simulink model "CSEI_HIL"  (R2020b)
settings: Solver=FixedStepAuto  StartTime=0.0  StopTime=Inf  FixedStep=0.01  RelTol=1e-3  EnableMultiTasking=on
undefined symbols (not defined in the file): X, Y, Z
libraries: robotlib x6, simulink x3
settings Model: Creator=erlendbasso  LastModifiedBy=erlendbasso
settings SolverCC: PositivePriorityOrder=on
settings OptimizationCC: EnhancedBackFolding=on  PassReuseOutputArgsAs=Individual arguments  ZeroExternalMemoryAtStartup=off  ZeroInternalMemoryAtStartup=off  MaxStackSize=64  OptimizeBlockOrder=speed  DifferentSizesBufferReuse=on  OptimizationCustomize=off  EfficientTunableParamExpr=on
settings DebuggingCC: ParameterTunabilityLossMsg=error
settings HardwareCC: ProdBitPerPointer=32  ProdBitPerSizeT=32  ProdBitPerPtrDiffT=32  ProdLargestAtomicInteger=Long  ProdLargestAtomicFloat=Double  ProdWordSize=32  ProdHWDeviceType=ARM Compatible->ARM Cortex
settings RTWCC: Description=Embedded Coder  SystemTargetFile=ert.tlc  HardwareBoard=Raspberry Pi - Robot Operating System (ROS)  TLCOptions="-aInlineSetEventsForThisBaseRateFcn=TLC_FALSE -aSuppressMultiTaskScheduler=TLC_FALSE  -aRateBasedStepFcn=0"  TemplateMakefile=ert_default_tmf  Toolchain=Catkin  TargetLang=C++
settings CodeAppCC: ForceParamTrailComments=on  IgnoreCustomStorageClasses=off  OperatorAnnotations=on  SimulinkDataObjDesc=on  SFDataObjDesc=on  InsertBlockDesc=on
settings ERTTargetCC: SupportContinuousTime=on

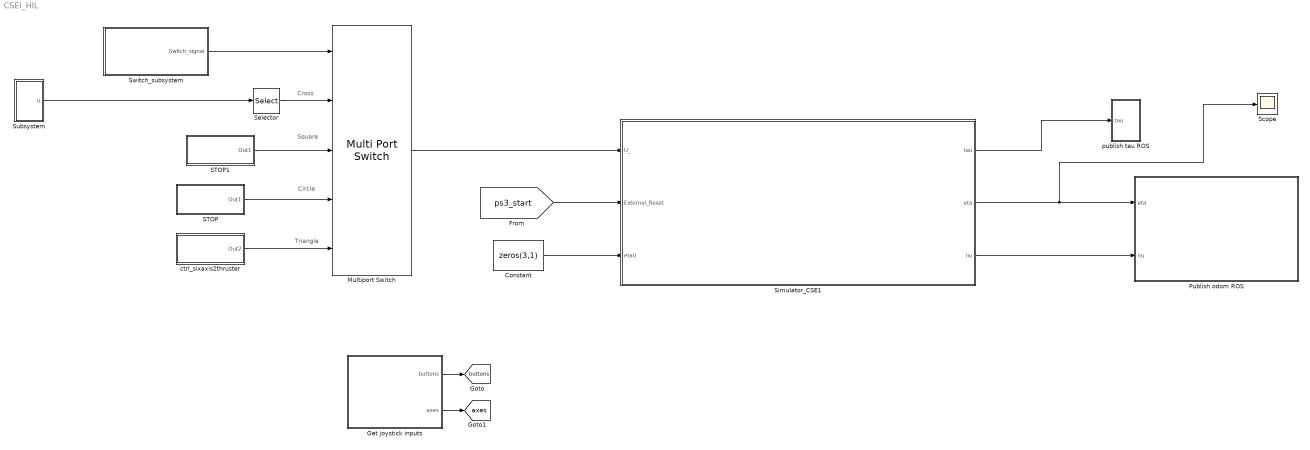
== system CSEI_HIL ==
  note: Square
  note: Triangle
  note: Circle
  note: Cross
  Constant : Constant  Value=zeros(3,1)
  Get joystick inputs : Subsystem
  Multiport Switch : MultiPortSwitch  Inputs=4
  Publish odom ROS : Subsystem
  STOP : Subsystem
  STOP1 : Subsystem
  Scope : Scope
  Selector : Selector  InputPortWidth=128  IndexOptions=Index vector (dialog)  Indices=[1:5]  OutputSizes=1
  Simulator_CSE1 : Subsystem
  Subsystem : Subsystem
  Switch_subsystem : Subsystem
  ctrl_sixaxis2thruster : Subsystem
  publish tau ROS : Subsystem
  tag scope: axes=global, buttons=global
  wires:
  Subsystem/1(u) -> Selector/1
  Switch_subsystem/1(Switch_signal) -> Multiport Switch/1
  ctrl_sixaxis2thruster/1(Out2) -> Multiport Switch/5
  STOP1/1(Out1) -> Multiport Switch/3
  STOP/1(Out1) -> Multiport Switch/4
  Get joystick inputs/1(buttons) -> [buttons]
  Get joystick inputs/2(axes) -> [axes]
  Constant/1 -> Simulator_CSE1/3(eta0)
  Simulator_CSE1/1(tau) -> publish tau ROS/1(tau)
  Simulator_CSE1/2(eta) -> Scope/1, Publish odom ROS/1(eta)
  Simulator_CSE1/3(nu) -> Publish odom ROS/2(nu)
  [ps3_start] -> Simulator_CSE1/2(External_Reset)
  Multiport Switch/1 -> Simulator_CSE1/1(U_)
  Selector/1 -> Multiport Switch/2

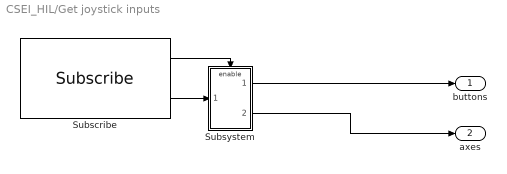
== system CSEI_HIL/Get joystick inputs ==
  Subscribe : robotlib/Subscribe  topicSource=Specify your own  topic=/joy  messageType=sensor_msgs/Joy  SampleTime=0.01  legacyBusStruct=off  messageQueueLength=1
  Subsystem : Subsystem
  buttons : Outport
  axes : Outport  Port=2
  wires:
  Subscribe/1 -> Subsystem/Enable
  Subscribe/2 -> Subsystem/1(In1)
  Subsystem/1(<Buttons>) -> buttons/1
  Subsystem/2(<Axes>) -> axes/1

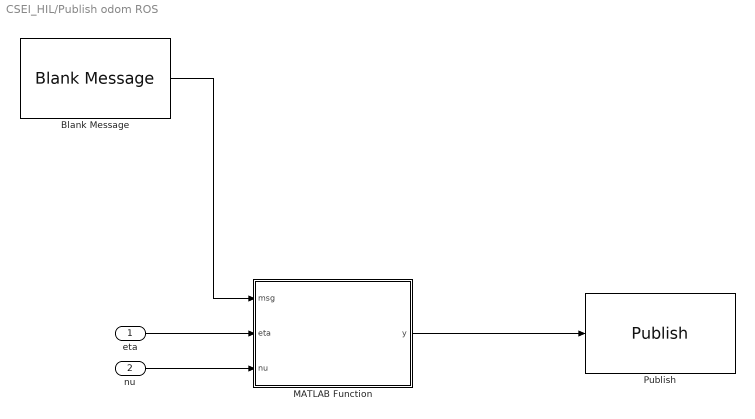
== system CSEI_HIL/Publish odom ROS ==
  eta : Inport
  nu : Inport  Port=2
  Blank Message : robotlib/Blank Message  messageClass=Message  entityType=nav_msgs/Odometry  messageType=nav_msgs/Odometry  SampleTime=0.01  legacyBusStruct=off
  MATLAB Function : MATLAB Function  TreatAsAtomicUnit=on
  Publish : robotlib/Publish  topicSource=Specify your own  topic=/qualisys/CSEI/odom  messageType=nav_msgs/Odometry  legacyBusStruct=off  messageQueueLength=1
  wires:
  MATLAB Function/1(y) -> Publish/1
  Blank Message/1 -> MATLAB Function/1(msg)
  eta/1 -> MATLAB Function/2(eta)
  nu/1 -> MATLAB Function/3(nu)

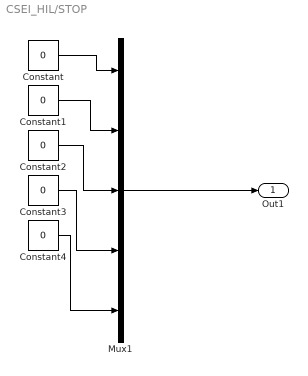
== system CSEI_HIL/STOP ==
  Constant{,1..4} (5 alike) : Constant  Value=0
  Mux1 : Mux  Inputs=5
  Out1 : Outport
  wires:
  Mux1/1 -> Out1/1
  Constant/1 -> Mux1/1
  Constant1/1 -> Mux1/2
  Constant2/1 -> Mux1/3
  Constant3/1 -> Mux1/4
  Constant4/1 -> Mux1/5

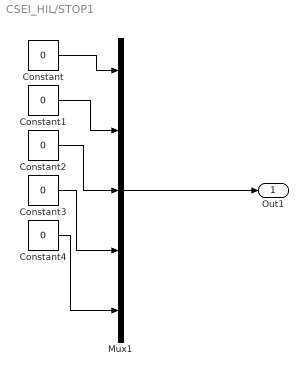
== system CSEI_HIL/STOP1 ==
  Constant{,1..4} (5 alike) : Constant  Value=0
  Mux1 : Mux  Inputs=5
  Out1 : Outport
  wires:
  Mux1/1 -> Out1/1
  Constant/1 -> Mux1/1
  Constant1/1 -> Mux1/2
  Constant2/1 -> Mux1/3
  Constant3/1 -> Mux1/4
  Constant4/1 -> Mux1/5

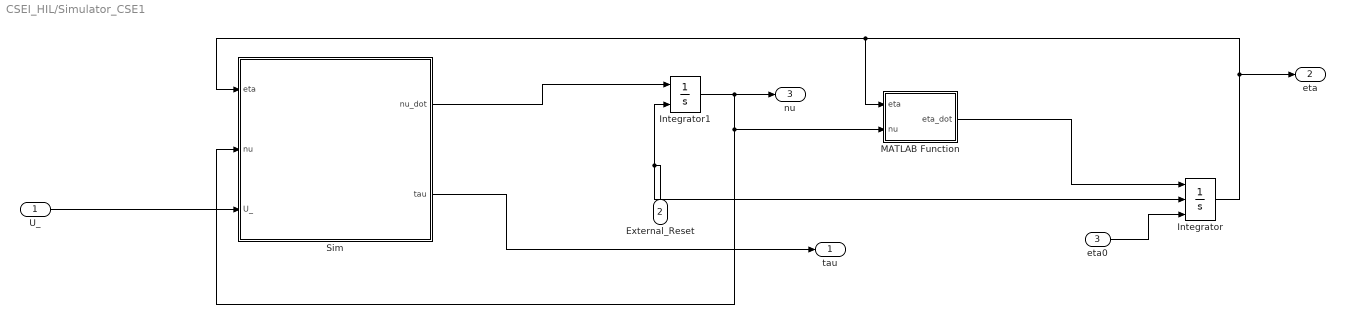
== system CSEI_HIL/Simulator_CSE1 ==
  U_ : Inport
  External_Reset : Inport  Port=2
  eta0 : Inport  Port=3
  Integrator : Integrator  ExternalReset=rising  InitialConditionSource=external  WrapState=on  WrappedStateUpperValue=[Inf;inf;pi]  WrappedStateLowerValue=[-Inf;-Inf;-pi]
  Integrator1 : Integrator  ExternalReset=rising  InitialCondition=zeros(3,1)
  MATLAB Function : MATLAB Function  TreatAsAtomicUnit=on
  Sim : MATLAB Function  TreatAsAtomicUnit=on
  tau : Outport
  eta : Outport  Port=2
  nu : Outport  Port=3
  wires:
  U_/1 -> Sim/3(U_)
  eta0/1 -> Integrator/3
  Sim/1(nu_dot) -> Integrator1/1
  External_Reset/1 -> Integrator/2, Integrator1/2
  Integrator1/1 -> MATLAB Function/2(nu), Sim/2(nu), nu/1
  Integrator/1 -> Sim/1(eta), MATLAB Function/1(eta), eta/1
  Sim/2(tau) -> tau/1
  MATLAB Function/1(eta_dot) -> Integrator/1

== system CSEI_HIL/Subsystem ==
  Bus Selector1 : BusSelector  OutputSignals=Data
  Subscribe : robotlib/Subscribe  topicSource=Specify your own  topic=/CSEI/u  messageType=std_msgs/Float64MultiArray  SampleTime=0.01  legacyBusStruct=off  messageQueueLength=1
  Subsystem1 : Subsystem
  u : Outport
  wires:
  Subscribe/1 -> Subsystem1/Enable
  Subscribe/2 -> Bus Selector1/1
  Subsystem1/1(Out1) -> u/1
  Bus Selector1/1 -> Subsystem1/1(<data>)  "<Data>"

== system CSEI_HIL/Switch_subsystem ==
  Memory : Memory  InitialCondition=4
  Switch_function : MATLAB Function  TreatAsAtomicUnit=on
  Switch_signal : Outport
  wires:
  Memory/1 -> Switch_function/2(temp)
  Switch_function/1(switch_signal) -> Switch_signal/1, Memory/1
  [buttons] -> Switch_function/1(buttons)

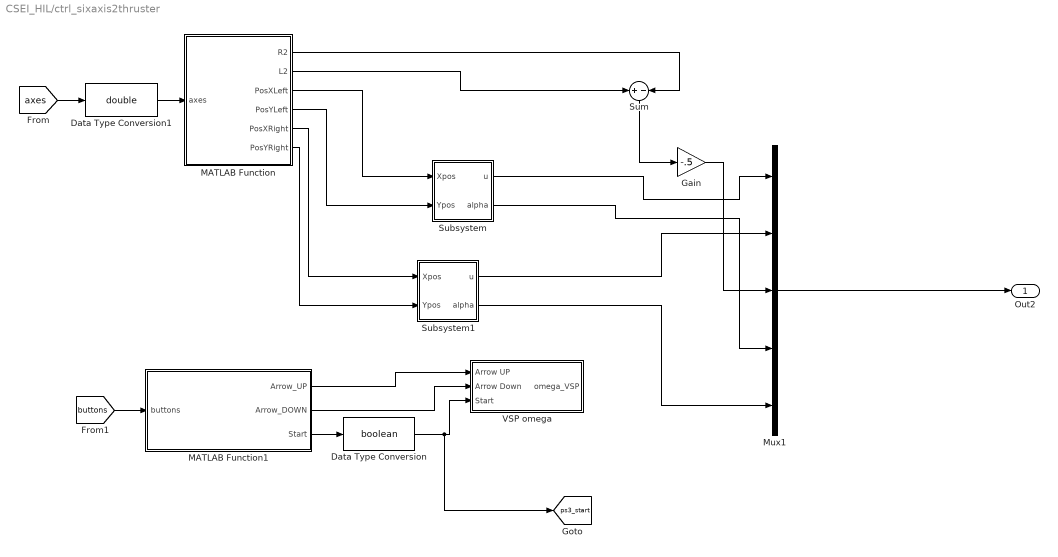
== system CSEI_HIL/ctrl_sixaxis2thruster ==
  Data Type Conversion : DataTypeConversion  OutDataTypeStr=boolean
  Data Type Conversion1 : DataTypeConversion  OutDataTypeStr=double
  Gain : Gain  Gain=-.5
  MATLAB Function : MATLAB Function  TreatAsAtomicUnit=on
  MATLAB Function1 : MATLAB Function  TreatAsAtomicUnit=on
  Mux1 : Mux  Inputs=5
  Subsystem : Subsystem
  Subsystem1 : Subsystem
  Sum : Sum  Inputs=+|-
  VSP omega : Subsystem
  Out2 : Outport
  tag scope: ps3_start=global
  wires:
  Mux1/1 -> Out2/1
  Subsystem/2(alpha) -> Mux1/4
  Subsystem1/2(alpha) -> Mux1/5
  MATLAB Function/1(R2) -> Sum/2
  Sum/1 -> Gain/1
  MATLAB Function/2(L2) -> Sum/1
  [axes] -> Data Type Conversion1/1
  MATLAB Function/3(PosXLeft) -> Subsystem/1(Xpos)
  MATLAB Function/4(PosYLeft) -> Subsystem/2(Ypos)
  MATLAB Function/5(PosXRight) -> Subsystem1/1(Xpos)
  MATLAB Function/6(PosYRight) -> Subsystem1/2(Ypos)
  [buttons] -> MATLAB Function1/1(buttons)
  MATLAB Function1/1(Arrow_UP) -> VSP omega/1(Arrow UP)
  MATLAB Function1/2(Arrow_DOWN) -> VSP omega/2(Arrow Down)
  MATLAB Function1/3(Start) -> Data Type Conversion/1
  Data Type Conversion/1 -> [ps3_start], VSP omega/3(Start)
  Data Type Conversion1/1 -> MATLAB Function/1(axes)
  Subsystem/1(u) -> Mux1/1
  Subsystem1/1(u) -> Mux1/2
  Gain/1 -> Mux1/3

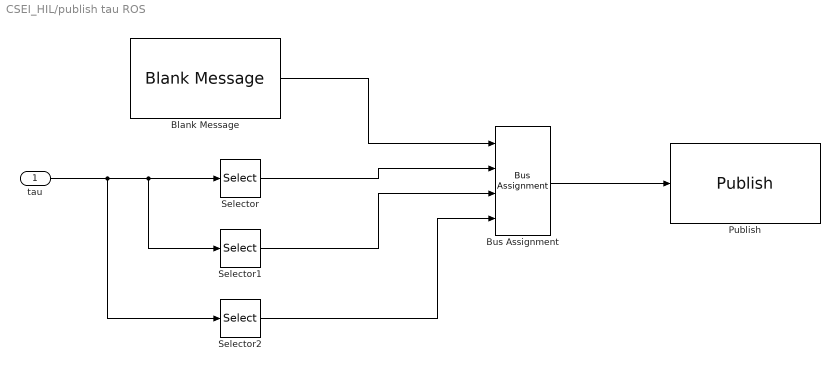
== system CSEI_HIL/publish tau ROS ==
  tau : Inport
  Blank Message : robotlib/Blank Message  messageClass=Message  entityType=geometry_msgs/Vector3  messageType=geometry_msgs/Vector3  SampleTime=0.01  legacyBusStruct=off
  Bus Assignment : BusAssignment  AssignedSignals=X,Y,Z
  Publish : robotlib/Publish  topicSource=Specify your own  topic=/CSEI/tau  messageType=geometry_msgs/Vector3  legacyBusStruct=off  messageQueueLength=1
  Selector : Selector  InputPortWidth=3  IndexOptions=Index vector (dialog)  Indices=[1]  OutputSizes=1
  Selector1 : Selector  InputPortWidth=3  IndexOptions=Index vector (dialog)  Indices=[2]  OutputSizes=1
  Selector2 : Selector  InputPortWidth=3  IndexOptions=Index vector (dialog)  Indices=[3]  OutputSizes=1
  wires:
  Bus Assignment/1 -> Publish/1
  Blank Message/1 -> Bus Assignment/1
  tau/1 -> Selector2/1, Selector1/1, Selector/1
  Selector/1 -> Bus Assignment/2
  Selector1/1 -> Bus Assignment/3
  Selector2/1 -> Bus Assignment/4

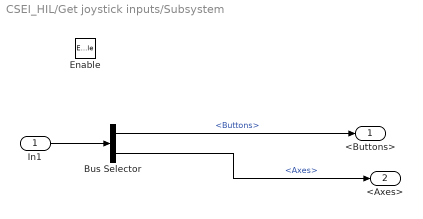
== system CSEI_HIL/Get joystick inputs/Subsystem ==
  In1 : Inport
  Enable : EnablePort
  Bus Selector : BusSelector  OutputSignals=Buttons,Axes
  <Buttons> : Outport
  <Axes> : Outport  Port=2
  wires:
  In1/1 -> Bus Selector/1
  Bus Selector/1 -> <Buttons>/1  "<Buttons>"
  Bus Selector/2 -> <Axes>/1  "<Axes>"

== system CSEI_HIL/Subsystem/Subsystem1 ==
  <data> : Inport
  Enable : EnablePort
  Bus to Vector : BusToVector
  Out1 : Outport
  wires:
  Bus to Vector/1 -> Out1/1
  <data>/1 -> Bus to Vector/1

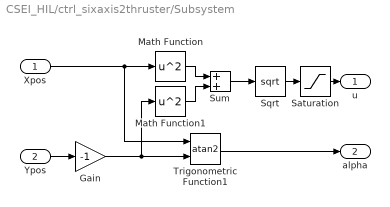
== system CSEI_HIL/ctrl_sixaxis2thruster/Subsystem ==
  Xpos : Inport
  Ypos : Inport  Port=2
  Gain : Gain  Gain=-1
  Math Function : Math  Operator=square  SignedPower=on  SaturateOnIntegerOverflow=on
  Math Function1 : Math  Operator=square  SignedPower=on  SaturateOnIntegerOverflow=on
  Saturation : Saturate  UpperLimit=1  LowerLimit=-1
  Sqrt : Sqrt  SaturateOnIntegerOverflow=on
  Sum : Sum
  Trigonometric Function1 : Trigonometry  Operator=atan2
  u : Outport
  alpha : Outport  Port=2
  wires:
  Xpos/1 -> Math Function/1, Trigonometric Function1/1
  Gain/1 -> Math Function1/1, Trigonometric Function1/2
  Trigonometric Function1/1 -> alpha/1
  Ypos/1 -> Gain/1
  Sum/1 -> Sqrt/1
  Math Function/1 -> Sum/1
  Math Function1/1 -> Sum/2
  Sqrt/1 -> Saturation/1
  Saturation/1 -> u/1

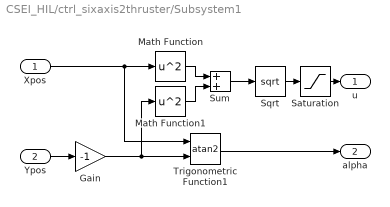
== system CSEI_HIL/ctrl_sixaxis2thruster/Subsystem1 ==
  Xpos : Inport
  Ypos : Inport  Port=2
  Gain : Gain  Gain=-1
  Math Function : Math  Operator=square  SignedPower=on  SaturateOnIntegerOverflow=on
  Math Function1 : Math  Operator=square  SignedPower=on  SaturateOnIntegerOverflow=on
  Saturation : Saturate  UpperLimit=1  LowerLimit=-1
  Sqrt : Sqrt  SaturateOnIntegerOverflow=on
  Sum : Sum
  Trigonometric Function1 : Trigonometry  Operator=atan2
  u : Outport
  alpha : Outport  Port=2
  wires:
  Xpos/1 -> Math Function/1, Trigonometric Function1/1
  Gain/1 -> Math Function1/1, Trigonometric Function1/2
  Trigonometric Function1/1 -> alpha/1
  Ypos/1 -> Gain/1
  Sum/1 -> Sqrt/1
  Math Function/1 -> Sum/1
  Math Function1/1 -> Sum/2
  Sqrt/1 -> Saturation/1
  Saturation/1 -> u/1

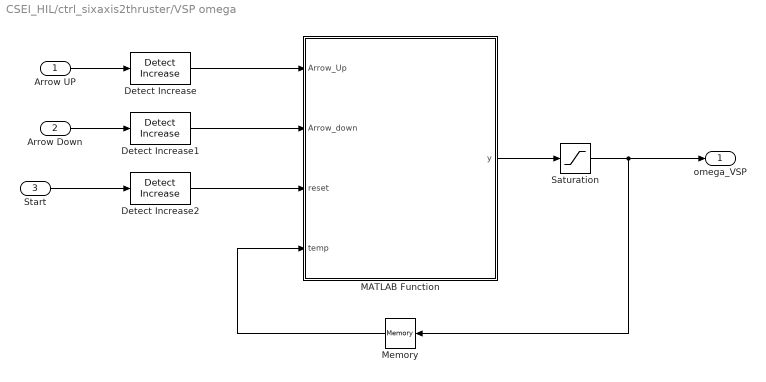
== system CSEI_HIL/ctrl_sixaxis2thruster/VSP omega ==
  Arrow UP : Inport
  Arrow Down : Inport  Port=2
  Start : Inport  Port=3
  Detect Increase : simulink/Logic and Bit Operations/Detect Increase  vinit=0.0  OutDataTypeStr=boolean
  Detect Increase1 : simulink/Logic and Bit Operations/Detect Increase  vinit=0.0  OutDataTypeStr=boolean
  Detect Increase2 : simulink/Logic and Bit Operations/Detect Increase  vinit=0.0  OutDataTypeStr=boolean
  MATLAB Function : MATLAB Function  TreatAsAtomicUnit=on
  Memory : Memory
  Saturation : Saturate  UpperLimit=0.8  LowerLimit=-0.8
  omega_VSP : Outport
  wires:
  Arrow UP/1 -> Detect Increase/1
  Arrow Down/1 -> Detect Increase1/1
  MATLAB Function/1(y) -> Saturation/1
  Memory/1 -> MATLAB Function/4(temp)
  Detect Increase/1 -> MATLAB Function/1(Arrow_Up)
  Detect Increase1/1 -> MATLAB Function/2(Arrow_down)
  Start/1 -> Detect Increase2/1
  Detect Increase2/1 -> MATLAB Function/3(reset)
  Saturation/1 -> omega_VSP/1, Memory/1

== matlab function CSEI_HIL/ctrl_sixaxis2thruster/MATLAB Function ==
  data: R2 output; axes input; L2 output; PosXLeft output; PosYLeft output; PosXRight output; PosYRight output
function [R2,L2,PosXLeft,PosYLeft,PosXRight,PosYRight] = fcn(axes)

% DualShock 3
% L2 = axes(9);
% R2 = axes(10);

% DualShock 4
L2 = axes(5);
R2 = axes(6);


PosXLeft = -axes(2);
PosYLeft = axes(1);

PosXRight = -axes(4);
PosYRight = axes(3);

== matlab function CSEI_HIL/ctrl_sixaxis2thruster/VSP omega/MATLAB Function ==
  data: Arrow_Up input; y output; Arrow_down input; reset input; temp input
function y = fcn(Arrow_Up,Arrow_down,reset,temp)
%#codegen
persistent signal;

signal = temp;

if Arrow_Up ~= 0
    signal = signal + 0.1;
end

if Arrow_down ~= 0
    signal = signal - 0.1;
end
 
if reset
    signal = double(0);
end



y = signal;

== matlab function CSEI_HIL/ctrl_sixaxis2thruster/MATLAB Function1 ==
  data: Arrow_UP output; buttons input; Arrow_DOWN output; Start output
function [Arrow_UP, Arrow_DOWN, Start] = extract_buttons(buttons)

% Start = double(buttons(4));
% Arrow_UP = double(buttons(5));
% Arrow_DOWN = double(buttons(7));


% DualShock 4
Start = double(buttons(10));
Arrow_UP = double(buttons(16));
Arrow_DOWN = double(buttons(18));

== matlab function CSEI_HIL/Simulator_CSE1/MATLAB Function ==
  settings: sampleTime=0.01
  data: eta input; nu input; eta_dot output
function eta_dot = fcn(eta,nu)

psi = eta(3);

J = [cos(psi) -sin(psi)   0
     sin(psi)  cos(psi)   0
     0         0          1];

eta_dot = J*nu;

== matlab function CSEI_HIL/Switch_subsystem/Switch_function ==
  data: buttons input; switch_signal output; temp input
%% Function that takes in impulse button sigals [0,1] and sends out a 
% different signal depentent pn which button has been pressed

function switch_signal = fcn(buttons,temp)
%#codegen
persistent signal;

% DualShock 3
% Triangle = buttons(13);
% Circle = buttons(14);
% Cross = buttons(15);
% Square = buttons(16);

% DualShock 4
Triangle = buttons(2);
Circle = buttons(3);
Cross = buttons(4);
Square = buttons(1);

signal = temp;

if Cross ~= 0
    signal = 1;
end

if Square ~= 0
    signal = 2;
end

if Circle ~= 0
    signal = 3;
end
    
if Triangle ~= 0
    signal = 4; 
end

switch_signal = signal;

== matlab function CSEI_HIL/Publish odom ROS/MATLAB Function ==
  data: msg input; eta input; y output Bus: SL_Bus_CSEI_HIL_nav_msgs_Odometry; nu input
function y = fcn(msg,eta,nu)

y = msg;

quat = eul2quat([0 0 eta(3)], 'XYZ');

y.Pose.Pose.Position.X = eta(1);
y.Pose.Pose.Position.Y = eta(2);
y.Pose.Pose.Position.Z = 0;
y.Pose.Pose.Orientation.W = quat(1);
y.Pose.Pose.Orientation.X = quat(2);
y.Pose.Pose.Orientation.Y = quat(3);
y.Pose.Pose.Orientation.Z = quat(4);


y.Twist.Twist.Linear.X = nu(1);
y.Twist.Twist.Linear.Y = nu(2);
y.Twist.Twist.Linear.Z = 0;
y.Twist.Twist.Angular.X = 0;
y.Twist.Twist.Angular.Y = 0;
y.Twist.Twist.Angular.Z = nu(3);

== matlab function CSEI_HIL/Simulator_CSE1/Sim ==
  settings: sampleTime=0.01
  data: eta input; nu input; U_ input; nu_dot output; tau output
function [nu_dot,tau] = fcn(eta,nu,U_)

u     = U_(1:3);
alpha = U_(4:5);

c1 = cos(alpha(1));
c2 = cos(alpha(2));
c3 = 0;
s1 = sin(alpha(1));
s2 = sin(alpha(2));
s3 = 1;

lx1 = -0.4574;
lx2 = -0.4574;
lx3 =  0.3875;
ly1 = -0.055;
ly2 =  0.055;
ly3 =  0;

k1 = 1.03;
k2 = 1.03;
k3 = 2.629;

B = [c1,              c2,              c3;
     s1,              s2,              s3;
     lx1*s1 - ly1*c1, lx2*s2 - ly2*c2, lx3*s3 - ly3*c3];


K = diag([k1,k2,k3]);
tau = B*K*u;

psi = eta(3);

J = [cos(psi) -sin(psi)   0
     sin(psi)  cos(psi)   0
     0         0          1];

% eta_dot = J*nu;

nu_1   = nu(1);
v   = nu(2);
r   = nu(3);

%% MATRICES 
%changed m from 14.79 to 14.11

m    = 14.11;   I_z  =  1.7600;   x_g = 0.0375;       % x_g  =  0.0460; % Table B.1

%% Added mass
%changed Y_vd from -1.0 to -10.0
X_ud  =     -2.0;											% Table B.1
					Y_vd =      -10.0;	N_vd =    -0.0;		% Table B.1
					Y_rd =      -0.0;	N_rd =    -1.0;		% Table B.1

%% Total mass matrix
m_11 = m-X_ud;
m_22 = m-Y_vd;
m_23 = m*x_g-Y_rd;
m_32 = m*x_g-N_vd; % noted as Y_rd in handbook, but same value
m_33 = I_z-N_rd;
% 
M    = [m_11 0    0
        0    m_22 m_23
        0    m_32 m_33];
% M   = [16, 0, 0; 0, 24, 0.53; 0, 0.53, 2.8];

	
%% Damping coefficients
% Comments at the end of the lines indicate the old values used.
X_u		= -0.6555;		X_v		= 0;
X_uu 	= 0.3545;		X_vv	= -2.443;
X_uuu 	= -3.787;		X_vvv	= 0;

						Y_v		= -1.33; 			Y_r		= -2.8; % Y_r
						Y_vv	= -2.776;			Y_rr	= -3.450; % Y_rr
						Y_vvv	= -64.91;			Y_rrr	= 0;
						
						Y_rv	= -0.805;			Y_vr	= -0.845; % Y_rv, Y_vr

						N_v		= 0;				N_r		= -1.900; % N_r
						N_vv	= -0.2088;			N_rr	= -0.750; % N_rr
						N_vvv	= 0;				N_rrr	= 0;
						
						N_rv	= 0.130;			N_vr	= 0.080; % N_rv, N_vr

%% Correolis matrix
c_13 = -(m-Y_vd)*v-(m*x_g-Y_rd)*r;
c_23 = (m-X_ud)*nu_1;
% C    = [0     0     c_13
%         0     0     c_23
%         -c_13 -c_23 0   ];
C = zeros(3,3);

%% Assembly of the damping matrix
%should be abs(u), abs(v) some places, only positive values? 

d_11 = -X_u - X_uu*abs(nu_1) - X_uuu*nu_1^2;
d_22 = -Y_v - Y_vv*abs(v) - Y_vvv*v^2 - Y_rv*abs(r);
d_33 = -N_r - N_rr*abs(r) - N_rrr*r^2 - N_vr*abs(v); % using abs(r)
%d_12 = -X_v - X_vv*v - X_vvv*v^2;
d_23 = -Y_r - Y_rr*abs(r) - Y_rrr*r^2 - Y_vr*abs(v);
d_32 = -N_v - N_vv*abs(v) - N_vvv*v^2 - N_rv*abs(r);

%D    = [d_11 d_12 0      vet ikke hvorfor d_12 er her
%        0    d_22 d_23
%        0    d_32 d_33];
D    = [d_11 0 0
        0    d_22 d_23
        0    d_32 d_33];

% D = [0.66 0 0; 0 1.3 2.8; 0 0 1.9];

%% CALCULATION
nu_dot = M\(tau-(C+D)*nu);

end
